simulink model "problem1model"  (R2020a)
settings: Solver=VariableStepAuto  StartTime=0.0  StopTime=10.0  RelTol=1e-3
PostLoadFcn:
  | K1=50;
  | M1=100;
  | b=50;
model workspace (MAT data in the model file):
  K12 = 1000
  M2 = 10
settings Model: OrderedModelArguments=off  Creator=Jake  LastModifiedBy=Jake

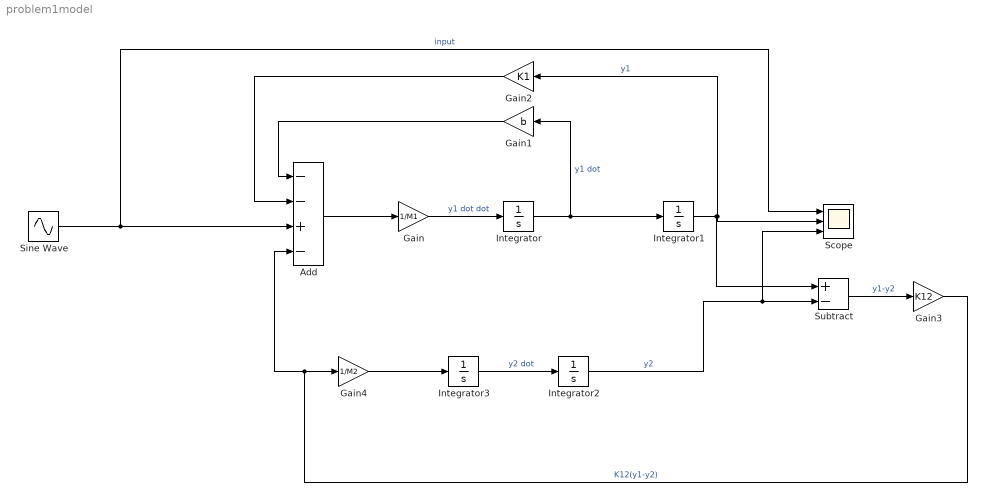
== system problem1model ==
  Add : Sum  Inputs=--+-
  Gain : Gain  Gain=1/M1
  Gain1 : Gain  Gain=b
  Gain2 : Gain  Gain=K1
  Gain3 : Gain  Gain=K12
  Gain4 : Gain  Gain=1/M2
  Integrator{,1..3} (4 alike) : Integrator
  Scope : Scope  NumInputPorts=3
  Sine Wave : Sin  Amplitude=2  Frequency=10  SampleTime=0.01
  Subtract : Sum  Inputs=+-
  wires:
  Add/1 -> Gain/1
  Gain/1 -> Integrator/1  "y1 dot dot"
  Integrator/1 -> Gain1/1, Integrator1/1  "y1 dot"
  Sine Wave/1 -> Scope/1, Add/3  "input"
  Gain1/1 -> Add/1
  Integrator1/1 -> Scope/2, Gain2/1, Subtract/1  "y1"
  Gain2/1 -> Add/2
  Integrator3/1 -> Integrator2/1  "y2 dot"
  Integrator2/1 -> Scope/3, Subtract/2  "y2"
  Subtract/1 -> Gain3/1  "y1-y2"
  Gain3/1 -> Add/4, Gain4/1  "K12(y1-y2)"
  Gain4/1 -> Integrator3/1
